simulink model "model"  (R2021b)
settings: Solver=VariableStepAuto  StartTime=0.0  StopTime=20000  RelTol=1e-3
values from neighbouring files (symbols this model uses):
  A = zeros(2)    [m1 — kopia.m]    (also in model.m)
  B = zeros(2)    [m1 — kopia.m]    (also in model.m)
  Cvg = Cpo*ROo*0.005    (= 14400)    [m1 — kopia.m]    (also in model.m = 14.4)
  Cvw = Cpp*ROp*60    (= 72360)    [m1 — kopia.m]    (also in model.m = 120600)
  dqg = 0 * qg0    (= 0)    [m1 — kopia.m]    (also in model.m = 200)
  dTzew = 3    [m1 — kopia.m]    (also in model.m = 0)
  init_con = [Twew0;Tg0]    [m1 — kopia.m]    (also in model.m = [Twew;Tg])
  Kcg = qg0/(Tg0-Twew0)    (= 100)    [m1 — kopia.m]    (also in model.m)
  Kcw = qg0/(Twew0-Tzew0)    (= 50)    [m1 — kopia.m]    (also in model.m)
  L1 = Kcg    (= 100)    [m1 — kopia.m]    (also in model.m)
  L2 = [Cvg*Kcw,Kcg*Kcw]    [m1 — kopia.m]    (also in model.m)
  L3 = [Cvw,Kcg+Kcw]    [m1 — kopia.m]    (also in model.m)
  L4 = Kcg*Kcw    (= 5000)    [m1 — kopia.m]    (also in model.m)
  M1 = [Cvw*Cvg,Cvg*(Kcg+Kcw)+Cvw*Kcg,Kcw*Kcg]    [m1 — kopia.m]    (also in model.m)
  qg0 = qgN * 1.0    (= 2000)    [m1 — kopia.m]    (also in model.m)
  stepTime = 1000    [m1 — kopia.m]    (also in model.m)
  Tg = 40    [model.m]
  Twew = 20    [model.m]
  Tzew0 = TzewN + 0    (= -20)    [m1 — kopia.m]    (also in model.m)
settings Model: Creator=Lab320  LastModifiedBy=rogow
settings SolverCC: AlgebraicLoopSolver=TrustRegion
settings DebuggingCC: SFMachineParentedDataDiag=warning

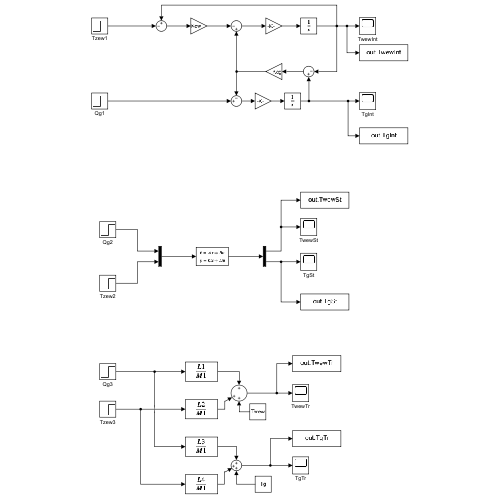
[thumbnail: Simulink's stored preview of the top-level diagram]
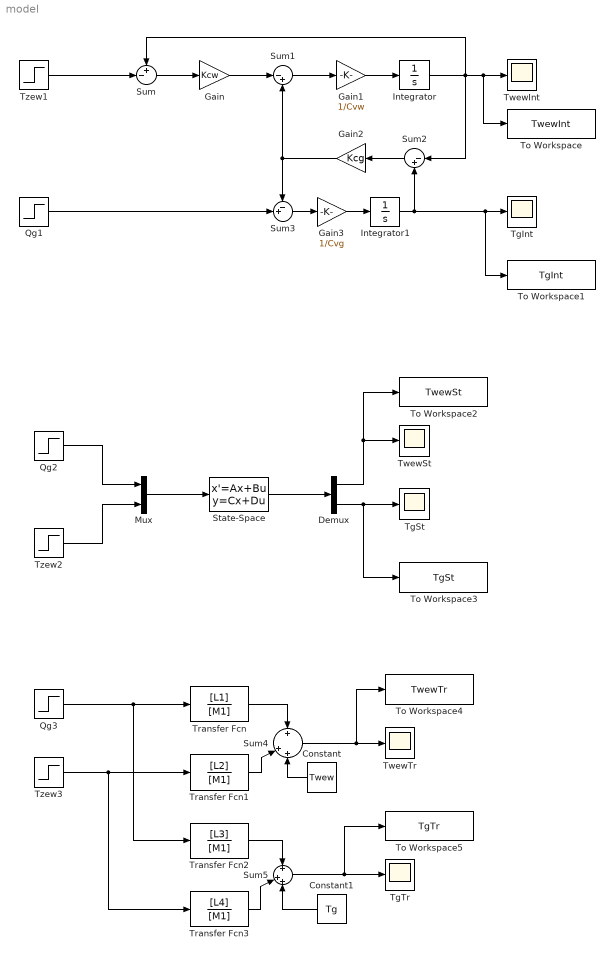
== system model ==
  Constant : Constant  Value=Twew
  Constant1 : Constant  Value=Tg
  Demux : Demux  Outputs=2
  Gain : Gain  Gain=Kcw
  Gain1 : Gain  Gain=1/Cvw
  Gain2 : Gain  Gain=Kcg
  Gain3 : Gain  Gain=1/Cvg
  Integrator : Integrator  InitialCondition=Twew
  Integrator1 : Integrator  InitialCondition=Tg
  Mux : Mux  Inputs=2
  Qg1 : Step  Time=stepTime  Before=qg0  After=qg0+dqg  SampleTime=0
  Qg2 : Step  Time=stepTime  Before=qg0  After=qg0+dqg  SampleTime=0
  Qg3 : Step  Time=stepTime  After=dqg  SampleTime=0
  State-Space : StateSpace  A=A  B=B  C=[1,0;0,1]  D=[0,0;0,0]  InitialCondition=init_con
  Sum : Sum  Inputs=+-|
  Sum1 : Sum  Inputs=|-+
  Sum2 : Sum  Inputs=|-+
  Sum3 : Sum  Inputs=-+|
  Sum4 : Sum  Inputs=+|++
  Sum5 : Sum  Inputs=+|++
  TgInt : Scope
  TgSt : Scope
  TgTr : Scope
  To Workspace : ToWorkspace  VariableName=TwewInt  SaveFormat=Timeseries  SampleTime=-1
  To Workspace1 : ToWorkspace  VariableName=TgInt  SaveFormat=Timeseries  SampleTime=-1
  To Workspace2 : ToWorkspace  VariableName=TwewSt  SaveFormat=Timeseries  SampleTime=-1
  To Workspace3 : ToWorkspace  VariableName=TgSt  SaveFormat=Timeseries  SampleTime=-1
  To Workspace4 : ToWorkspace  VariableName=TwewTr  SaveFormat=Timeseries  SampleTime=-1
  To Workspace5 : ToWorkspace  VariableName=TgTr  SaveFormat=Timeseries  SampleTime=-1
  Transfer Fcn : TransferFcn  Numerator=[L1]  Denominator=[M1]
  Transfer Fcn1 : TransferFcn  Numerator=[L2]  Denominator=[M1]
  Transfer Fcn2 : TransferFcn  Numerator=[L3]  Denominator=[M1]
  Transfer Fcn3 : TransferFcn  Numerator=[L4]  Denominator=[M1]
  TwewInt : Scope
  TwewSt : Scope
  TwewTr : Scope
  Tzew1 : Step  Time=stepTime  Before=Tzew0  After=Tzew0+dTzew  SampleTime=0
  Tzew2 : Step  Time=stepTime  Before=Tzew0  After=Tzew0+dTzew  SampleTime=0
  Tzew3 : Step  Time=stepTime  After=dTzew  SampleTime=0
  wires:
  Mux/1 -> State-Space/1
  State-Space/1 -> Demux/1
  Demux/1 -> TwewSt/1, To Workspace2/1
  Demux/2 -> To Workspace3/1, TgSt/1
  Qg2/1 -> Mux/1
  Tzew2/1 -> Mux/2
  Tzew1/1 -> Sum/2
  Sum/1 -> Gain/1
  Gain/1 -> Sum1/1
  Sum1/1 -> Gain1/1
  Gain1/1 -> Integrator/1
  Integrator/1 -> Sum2/1, Sum/1, To Workspace/1, TwewInt/1
  Sum2/1 -> Gain2/1
  Gain2/1 -> Sum3/1, Sum1/2
  Qg1/1 -> Sum3/2
  Sum3/1 -> Gain3/1
  Gain3/1 -> Integrator1/1
  Integrator1/1 -> To Workspace1/1, TgInt/1, Sum2/2
  Qg3/1 -> Transfer Fcn2/1, Transfer Fcn/1
  Tzew3/1 -> Transfer Fcn3/1, Transfer Fcn1/1
  Transfer Fcn/1 -> Sum4/1
  Transfer Fcn1/1 -> Sum4/2
  Transfer Fcn2/1 -> Sum5/1
  Transfer Fcn3/1 -> Sum5/2
  Sum4/1 -> To Workspace4/1, TwewTr/1
  Sum5/1 -> To Workspace5/1, TgTr/1
  Constant/1 -> Sum4/3
  Constant1/1 -> Sum5/3
